simulink model "from_sldv1"  (R2016a)
settings: Solver=VariableStepAuto  StartTime=0.0  StopTime=10.0  RelTol=1e-3
libraries: simulink x13, sldvlib x8
settings Model: Creator=Teme  LastModifiedBy=Teme

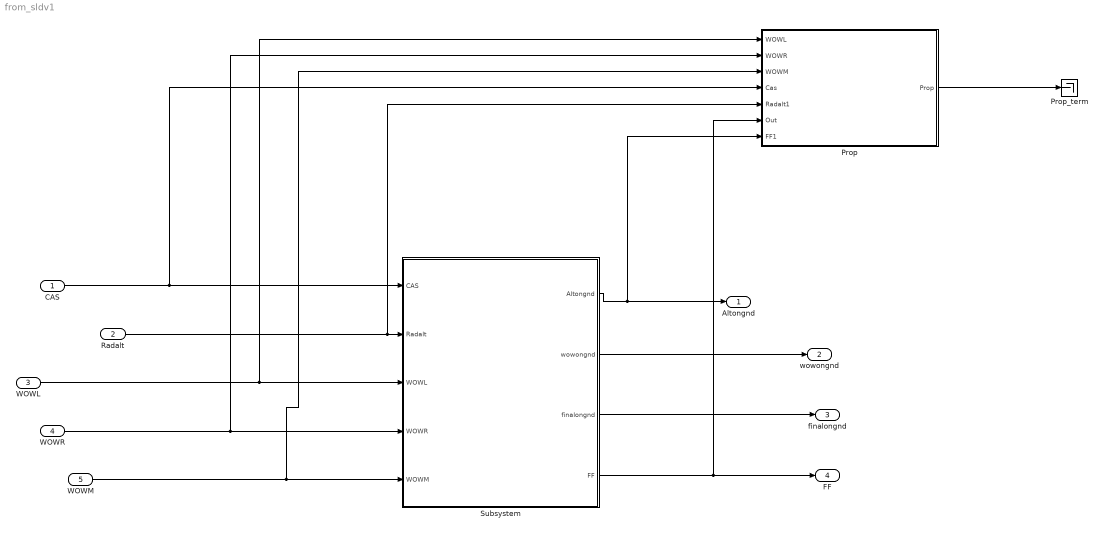
== system from_sldv1 ==
  CAS : Inport
  Radalt : Inport  Port=2
  WOWL : Inport  Port=3
  WOWR : Inport  Port=4
  WOWM : Inport  Port=5
  Prop : Subsystem  TreatAsAtomicUnit=on  mask(Observer){AnnotationType=ensures, ObserverType=[]}
      mask prompts: AnnotationType "Type of annotation (pre/post...)"; ObserverType "Observer type"
      mask help:
      | Set an observer for the system.
      | The annotation type parameter sets the type of observer:
      | - requires : pre-condition
      | - ensures : post-condition
      | - assert : an assertion
      | - observer : the observer computes a special type of properties
      mask TypeOptions AnnotationType: ensures | requires | assert | observer
      mask Callback AnnotationType:
      | paramStr = get_param(gcb, 'MaskValues');
      | if strcmp(paramStr{1}(1),'o')
      | set_param(gcb,'MaskVisibilities',{'on';'on'});
      | paramStr{2} = 'ellipsoid';
      | set_param(gcb,'MaskValues',paramStr);
      | else
      | set_param(gcb,'MaskVisibilities',{'on';'off'});
      | end
      | clear paramStr;
      mask Callback ObserverType:
      | paramStr = get_param(gcb, 'MaskValues');
      | if strcmp(paramStr{1}(1),'o')
      | set_param(gcb,'MaskVisibilities',{'on';'on'});
      | paramStr{2} = 'ellipsoid';
      | set_param(gcb,'MaskValues',paramStr);
      | else
      | set_param(gcb,'MaskVisibilities',{'on';'off'});
      | end
      | clear paramStr;
      mask Display:
      | color('red')
      | text(0.5, 0.5, ['CoCoSpec: ''' get_param(gcb,'name') ''''], 'horizontalAlignment', 'center');
      | text(0.99, 0.03, '{\bf\fontsize{12}TO BE VERIFIED}', 'hor', 'right', 'ver', 'bottom', 'texmode', 'on');
  Prop_term : Terminator
  Subsystem : Subsystem
  Altongnd : Outport
  wowongnd : Outport  Port=2
  finalongnd : Outport  Port=3
  FF : Outport  Port=4
  wires:
  CAS/1 -> Prop/4(Cas), Subsystem/1(CAS)
  Radalt/1 -> Prop/5(Radalt1), Subsystem/2(Radalt)
  WOWL/1 -> Subsystem/3(WOWL), Prop/1(WOWL)
  WOWR/1 -> Subsystem/4(WOWR), Prop/2(WOWR)
  WOWM/1 -> Subsystem/5(WOWM), Prop/3(WOWM)
  Subsystem/1(Altongnd) -> Prop/7(FF1), Altongnd/1
  Subsystem/2(wowongnd) -> wowongnd/1
  Subsystem/3(finalongnd) -> finalongnd/1
  Subsystem/4(FF) -> Prop/6(Out), FF/1
  Prop/1(Prop) -> Prop_term/1

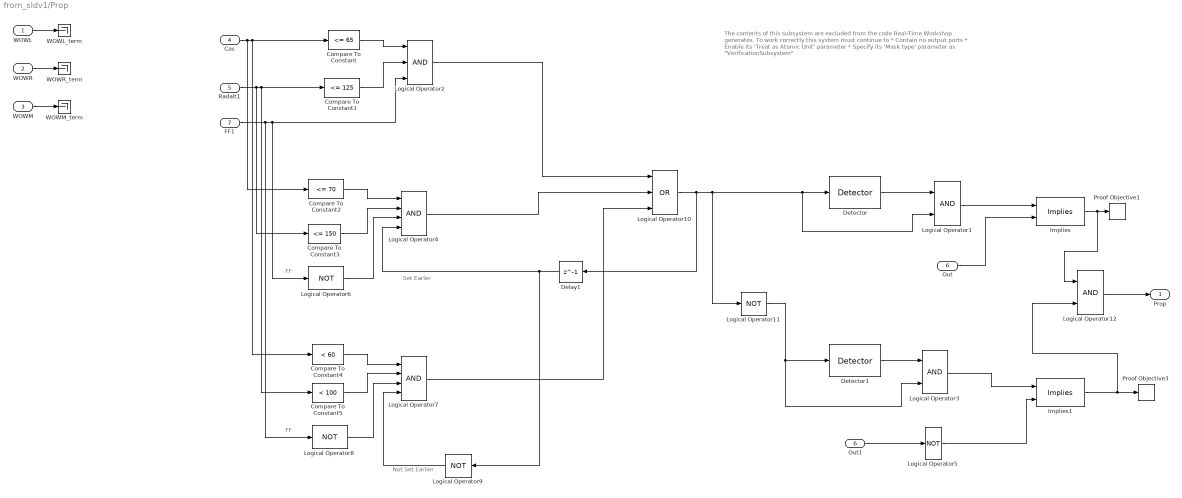
== system from_sldv1/Prop ==
  note: FF
  note: FF
  note: Not Set Earlier
  note: Set Earler
  note: The contents of this subsystem are excluded from the code Real-Time
      | Workshop generates.
      |
      | To work correctly this system must continue to
      | * Contain no output ports
      | * Enable its 'Treat as Atomic Unit' parameter
      | * Specify its 'Mask type' parameter as "VerificationSubsystem"
  WOWL : Inport
  WOWR : Inport  Port=2
  WOWM : Inport  Port=3
  Cas : Inport  Port=4
  Radalt1 : Inport  Port=5
  Out : Inport  Port=6
  FF1 : Inport  Port=7
  Compare To Constant : simulink/Logic and Bit Operations/Compare To Constant  relop=<=  const=65  OutDataTypeStr=boolean
  Compare To Constant1 : simulink/Logic and Bit Operations/Compare To Constant  relop=<=  const=125  OutDataTypeStr=boolean
  Compare To Constant2 : simulink/Logic and Bit Operations/Compare To Constant  relop=<=  const=70  OutDataTypeStr=boolean
  Compare To Constant3 : simulink/Logic and Bit Operations/Compare To Constant  relop=<=  const=150  OutDataTypeStr=boolean
  Compare To Constant4 : simulink/Logic and Bit Operations/Compare To Constant  relop=<  const=60  OutDataTypeStr=boolean
  Compare To Constant5 : simulink/Logic and Bit Operations/Compare To Constant  relop=<  const=100  OutDataTypeStr=boolean
  Delay1 : Delay  DelayLength=1  InitialCondition=0
  Detector : sldvlib/Temporal Operators/Detector  reset=off  typ=Synchronized  in_hold=21  delay=1  out_hold=3
  Detector1 : sldvlib/Temporal Operators/Detector  reset=off  typ=Synchronized  in_hold=41  delay=1  out_hold=3
  Implies : sldvlib/Verification Utilities/Implies
  Implies1 : sldvlib/Verification Utilities/Implies
  Logical Operator1 : Logic  AllPortsSameDT=off  OutDataTypeStr=boolean
  Logical Operator10 : Logic  Operator=OR  Inputs=3  AllPortsSameDT=off  OutDataTypeStr=boolean
  Logical Operator{5..6,8..9,11} (5 alike) : Logic  Operator=NOT  AllPortsSameDT=off  OutDataTypeStr=boolean
  Logical Operator12 : Logic  AllPortsSameDT=off  OutDataTypeStr=boolean
  Logical Operator2 : Logic  Inputs=3  AllPortsSameDT=off  OutDataTypeStr=boolean
  Logical Operator3 : Logic  AllPortsSameDT=off  OutDataTypeStr=boolean
  Logical Operator4 : Logic  Inputs=4  AllPortsSameDT=off  OutDataTypeStr=boolean
  Logical Operator7 : Logic  Inputs=4  AllPortsSameDT=off  OutDataTypeStr=boolean
  Out1 : InportShadow  Port=6
  Proof Objective1 : sldvlib/Objectives and Constraints/Proof Objective  enabled=on  customAVTBlockType=Proof Objective  intervals=true  dispValues=on  outEnabled=off  enableStopSim=on
      settings: AttributesFormatString=%<intervals>
  Proof Objective3 : sldvlib/Objectives and Constraints/Proof Objective  enabled=on  customAVTBlockType=Proof Objective  intervals=true  dispValues=on  outEnabled=off  enableStopSim=on
      settings: AttributesFormatString=%<intervals>
  WOWL_term : Terminator
  WOWM_term : Terminator
  WOWR_term : Terminator
  Prop : Outport
  wires:
  WOWL/1 -> WOWL_term/1
  WOWR/1 -> WOWR_term/1
  WOWM/1 -> WOWM_term/1
  Out/1 -> Implies/2
  Compare To Constant/1 -> Logical Operator2/1
  Compare To Constant1/1 -> Logical Operator2/2
  Implies/1 -> Logical Operator12/1, Proof Objective1/1
  Logical Operator3/1 -> Implies1/1
  Detector1/1 -> Logical Operator3/1
  Compare To Constant2/1 -> Logical Operator4/1
  Compare To Constant3/1 -> Logical Operator4/2
  Implies1/1 -> Logical Operator12/2, Proof Objective3/1
  Logical Operator5/1 -> Implies1/2
  Out1/1 -> Logical Operator5/1
  Logical Operator6/1 -> Logical Operator4/3
  Delay1/1 -> Logical Operator9/1, Logical Operator4/4
  Cas/1 -> Compare To Constant2/1, Compare To Constant4/1, Compare To Constant/1
  Radalt1/1 -> Compare To Constant3/1, Compare To Constant5/1, Compare To Constant1/1
  Compare To Constant4/1 -> Logical Operator7/1
  Compare To Constant5/1 -> Logical Operator7/2
  FF1/1 -> Logical Operator8/1, Logical Operator6/1, Logical Operator2/3
  Logical Operator8/1 -> Logical Operator7/3
  Logical Operator9/1 -> Logical Operator7/4
  Logical Operator2/1 -> Logical Operator10/1
  Logical Operator4/1 -> Logical Operator10/2
  Logical Operator7/1 -> Logical Operator10/3
  Logical Operator10/1 -> Delay1/1, Logical Operator1/2, Detector/1, Logical Operator11/1
  Detector/1 -> Logical Operator1/1
  Logical Operator1/1 -> Implies/1
  Logical Operator11/1 -> Logical Operator3/2, Detector1/1
  Logical Operator12/1 -> Prop/1

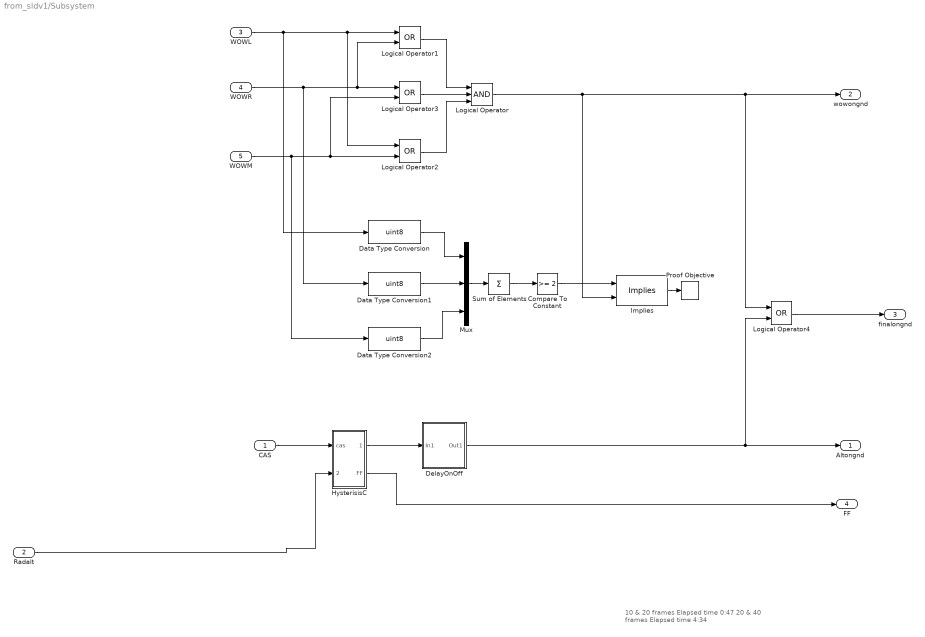
== system from_sldv1/Subsystem ==
  note: 10 & 20 frames Elapsed time 0:47
      | 20 & 40 frames Elapsed time 4:34
  CAS : Inport
  Radalt : Inport  Port=2
  WOWL : Inport  Port=3
  WOWR : Inport  Port=4
  WOWM : Inport  Port=5
  Compare To Constant : simulink/Logic and Bit Operations/Compare To Constant  relop=>=  const=2  OutDataTypeStr=boolean
  Data Type Conversion : DataTypeConversion  OutDataTypeStr=uint8
  Data Type Conversion1 : DataTypeConversion  OutDataTypeStr=uint8
  Data Type Conversion2 : DataTypeConversion  OutDataTypeStr=uint8
  DelayOnOff : Subsystem
  HysterisisC : Subsystem
  Implies : sldvlib/Verification Utilities/Implies
  Logical Operator : Logic  Inputs=3  AllPortsSameDT=off  OutDataTypeStr=boolean
  Logical Operator{1..4} (4 alike) : Logic  Operator=OR  AllPortsSameDT=off  OutDataTypeStr=boolean
  Mux : Mux  Inputs=3
  Proof Objective : sldvlib/Objectives and Constraints/Proof Objective  enabled=on  customAVTBlockType=Proof Objective  intervals=true  dispValues=on  outEnabled=off  enableStopSim=off
      settings: AttributesFormatString=%<intervals>
  Sum of Elements : Sum  Inputs=+
  Altongnd : Outport
  wowongnd : Outport  Port=2
  finalongnd : Outport  Port=3
  FF : Outport  Port=4
  wires:
  HysterisisC/1(Out1) -> DelayOnOff/1(In1)
  Logical Operator/1 -> Implies/2, wowongnd/1, Logical Operator4/1
  Data Type Conversion1/1 -> Mux/2
  Data Type Conversion2/1 -> Mux/3
  Data Type Conversion/1 -> Mux/1
  Mux/1 -> Sum of Elements/1
  Sum of Elements/1 -> Compare To Constant/1
  Compare To Constant/1 -> Implies/1
  Implies/1 -> Proof Objective/1
  Logical Operator4/1 -> finalongnd/1
  DelayOnOff/1(Out1) -> Altongnd/1, Logical Operator4/2
  Logical Operator1/1 -> Logical Operator/1
  WOWL/1 -> Logical Operator1/1, Logical Operator2/1, Data Type Conversion/1
  WOWR/1 -> Logical Operator3/1, Logical Operator1/2, Data Type Conversion1/1
  WOWM/1 -> Logical Operator2/2, Logical Operator3/2, Data Type Conversion2/1
  Logical Operator3/1 -> Logical Operator/2
  Logical Operator2/1 -> Logical Operator/3
  CAS/1 -> HysterisisC/1(cas)
  Radalt/1 -> HysterisisC/2(radalt)
  HysterisisC/2(FF) -> FF/1

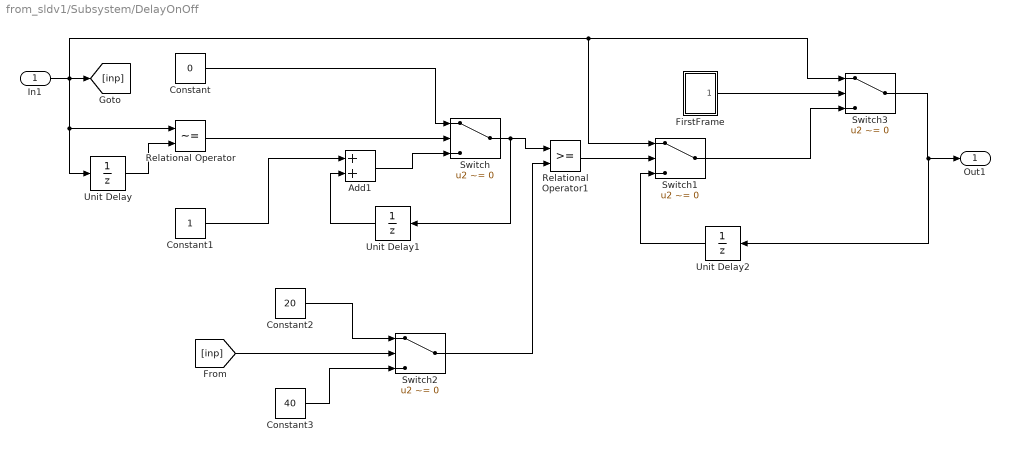
== system from_sldv1/Subsystem/DelayOnOff ==
  In1 : Inport
  Add1 : Sum
  Constant : Constant  Value=0
  Constant1 : Constant
  Constant2 : Constant  Value=20
  Constant3 : Constant  Value=40
  FirstFrame : Subsystem
  Relational Operator : RelationalOperator  Operator=~=  OutDataTypeStr=boolean
  Relational Operator1 : RelationalOperator  OutDataTypeStr=boolean
  Switch{,1..3} (4 alike) : Switch  Criteria=u2 ~= 0
  Unit Delay : UnitDelay  SampleTime=-1
  Unit Delay1 : UnitDelay  SampleTime=-1
  Unit Delay2 : UnitDelay  SampleTime=-1
  Out1 : Outport
  wires:
  Unit Delay1/1 -> Add1/2
  Constant2/1 -> Switch2/1
  Constant1/1 -> Add1/1
  Relational Operator/1 -> Switch/2
  Constant/1 -> Switch/1
  Unit Delay/1 -> Relational Operator/2
  Unit Delay2/1 -> Switch1/3
  Relational Operator1/1 -> Switch1/2
  Switch/1 -> Unit Delay1/1, Relational Operator1/1
  Constant3/1 -> Switch2/3
  Switch2/1 -> Relational Operator1/2
  Add1/1 -> Switch/3
  [inp] -> Switch2/2
  FirstFrame/1(Out1) -> Switch3/2
  In1/1 -> Switch3/1, Switch1/1, Unit Delay/1, Relational Operator/1, [inp]
  Switch1/1 -> Switch3/3
  Switch3/1 -> Unit Delay2/1, Out1/1

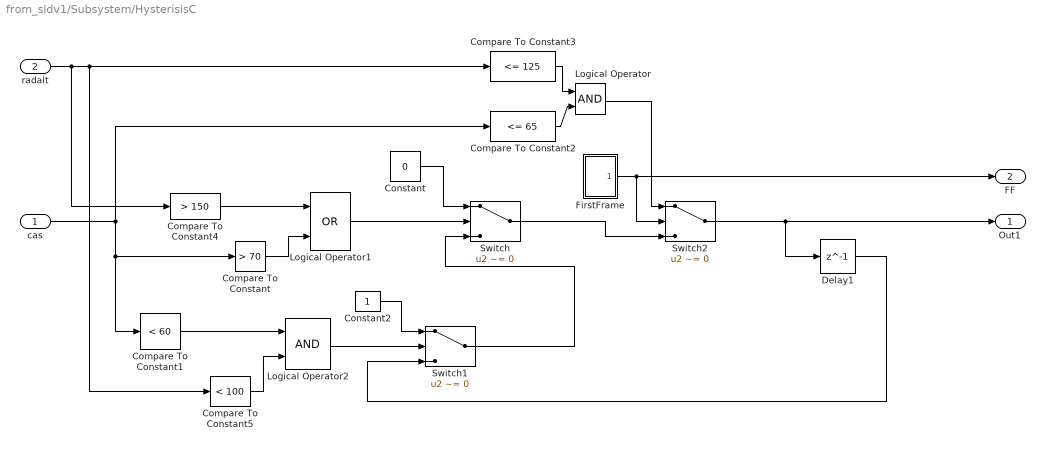
== system from_sldv1/Subsystem/HysterisisC ==
  cas : Inport
  radalt : Inport  Port=2
  Compare To Constant : simulink/Logic and Bit Operations/Compare To Constant  relop=>  const=70  OutDataTypeStr=boolean
  Compare To Constant1 : simulink/Logic and Bit Operations/Compare To Constant  relop=<  const=60  OutDataTypeStr=boolean
  Compare To Constant2 : simulink/Logic and Bit Operations/Compare To Constant  relop=<=  const=65  OutDataTypeStr=boolean
  Compare To Constant3 : simulink/Logic and Bit Operations/Compare To Constant  relop=<=  const=125  OutDataTypeStr=boolean
  Compare To Constant4 : simulink/Logic and Bit Operations/Compare To Constant  relop=>  const=150  OutDataTypeStr=boolean
  Compare To Constant5 : simulink/Logic and Bit Operations/Compare To Constant  relop=<  const=100  OutDataTypeStr=boolean
  Constant : Constant  Value=0
  Constant2 : Constant
  Delay1 : Delay  DelayLength=1  InitialCondition=0
  FirstFrame : Subsystem
  Logical Operator : Logic  AllPortsSameDT=off  OutDataTypeStr=boolean
  Logical Operator1 : Logic  Operator=OR  AllPortsSameDT=off  OutDataTypeStr=boolean
  Logical Operator2 : Logic  AllPortsSameDT=off  OutDataTypeStr=boolean
  Switch : Switch  Criteria=u2 ~= 0
  Switch1 : Switch  Criteria=u2 ~= 0
  Switch2 : Switch  Criteria=u2 ~= 0
  Out1 : Outport
  FF : Outport  Port=2
  wires:
  Switch1/1 -> Switch/3
  Delay1/1 -> Switch1/3
  cas/1 -> Compare To Constant1/1, Compare To Constant/1, Compare To Constant2/1
  Constant2/1 -> Switch1/1
  Switch/1 -> Switch2/3
  Constant/1 -> Switch/1
  FirstFrame/1(Out1) -> FF/1, Switch2/2
  Switch2/1 -> Out1/1, Delay1/1
  radalt/1 -> Compare To Constant4/1, Compare To Constant5/1, Compare To Constant3/1
  Compare To Constant3/1 -> Logical Operator/1
  Compare To Constant2/1 -> Logical Operator/2
  Logical Operator/1 -> Switch2/1
  Compare To Constant/1 -> Logical Operator1/2
  Compare To Constant4/1 -> Logical Operator1/1
  Logical Operator1/1 -> Switch/2
  Compare To Constant1/1 -> Logical Operator2/1
  Compare To Constant5/1 -> Logical Operator2/2
  Logical Operator2/1 -> Switch1/2

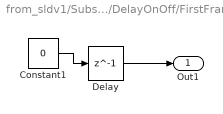
== system from_sldv1/Subsystem/DelayOnOff/FirstFrame ==
  Constant1 : Constant  Value=0
  Delay : Delay  DelayLength=1  InitialCondition=0
  Out1 : Outport
  wires:
  Constant1/1 -> Delay/1
  Delay/1 -> Out1/1

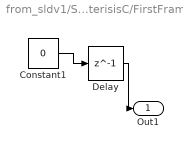
== system from_sldv1/Subsystem/HysterisisC/FirstFrame ==
  Constant1 : Constant  Value=0
  Delay : Delay  DelayLength=1  InitialCondition=1
  Out1 : Outport
  wires:
  Constant1/1 -> Delay/1
  Delay/1 -> Out1/1
